simulink model "sim_2"  (R2020a)
settings: Solver=VariableStepAuto  StartTime=0.0  StopTime=10  MaxStep=0.2  RelTol=1e-3
values from neighbouring files (symbols this model uses):
  k1 = 50    [parameters.m]
  k2 = 20    [parameters.m]
  q0 = [0, 0]'    [parameters.m]
libraries: simulink x1
settings Model: Creator=sirius  LastModifiedBy=sirius

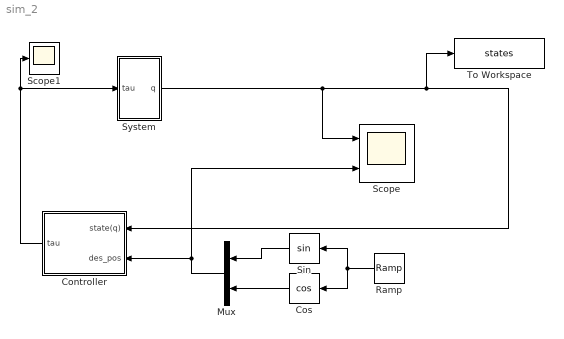
== system sim_2 ==
  Controller : Subsystem
  Cos : Trigonometry  Operator=cos
  Mux : Mux  Inputs=2
  Ramp : simulink/Sources/Ramp  slope=1  start=0  InitialOutput=0
  Scope : Scope  NumInputPorts=2
  Scope1 : Scope
  Sin : Trigonometry
  System : Subsystem
  To Workspace : ToWorkspace  VariableName=states  SampleTime=-1
  wires:
  Mux/1 -> Scope/2, Controller/2(des_pos)
  Controller/1(tau) -> Scope1/1, System/1(tau)
  System/1(q) -> Scope/1, To Workspace/1, Controller/1(state(q))
  Sin/1 -> Mux/1
  Cos/1 -> Mux/2
  Ramp/1 -> Sin/1, Cos/1

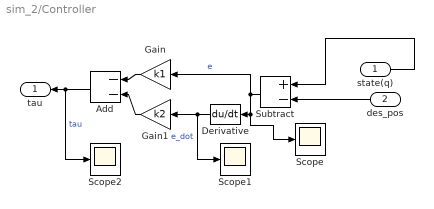
== system sim_2/Controller ==
  state(q) : Inport
  des_pos : Inport  Port=2
  Add : Sum  Inputs=--
  Derivative : Derivative
  Gain : Gain  Gain=k1
  Gain1 : Gain  Gain=k2
  Scope : Scope
  Scope1 : Scope
  Scope2 : Scope
  Subtract : Sum  Inputs=+-
  tau : Outport
  wires:
  Gain/1 -> Add/1
  state(q)/1 -> Subtract/1
  Gain1/1 -> Add/2
  Add/1 -> Scope2/1, tau/1  "tau"
  des_pos/1 -> Subtract/2
  Subtract/1 -> Gain/1, Scope/1, Derivative/1  "e"
  Derivative/1 -> Scope1/1, Gain1/1  "e_dot"

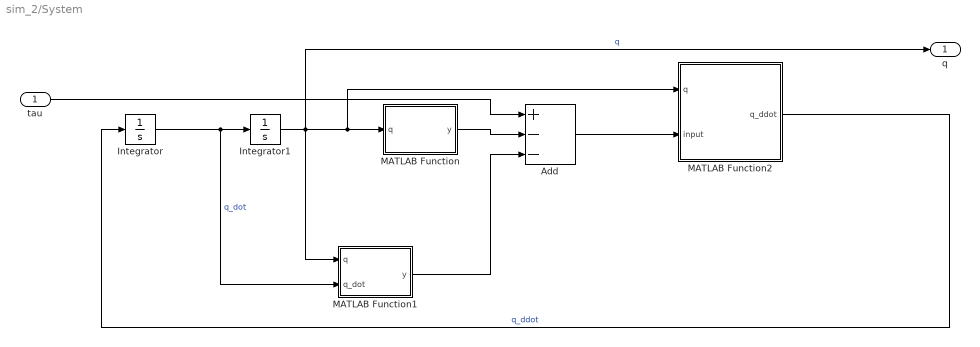
== system sim_2/System ==
  tau : Inport
  Add : Sum  Inputs=+--
  Integrator : Integrator  InitialCondition=q0
  Integrator1 : Integrator  InitialCondition=q0
  MATLAB Function : MATLAB Function  TreatAsAtomicUnit=on
  MATLAB Function1 : MATLAB Function  TreatAsAtomicUnit=on
  MATLAB Function2 : MATLAB Function  TreatAsAtomicUnit=on
  q : Outport
  wires:
  MATLAB Function1/1(y) -> Add/3
  Integrator1/1 -> MATLAB Function1/1(q), q/1, MATLAB Function2/1(q), MATLAB Function/1(q)  "q"
  tau/1 -> Add/1
  Integrator/1 -> MATLAB Function1/2(q_dot), Integrator1/1  "q_dot"
  MATLAB Function2/1(q_ddot) -> Integrator/1  "q_ddot"
  Add/1 -> MATLAB Function2/2(input)
  MATLAB Function/1(y) -> Add/2

== matlab function sim_2/System/MATLAB Function1 ==
  data: q input; y output; q_dot input
function y = V(q,q_dot)
y  = [-2*q_dot(1)*q_dot(2)*sin(q(2)) - (q_dot(2)^2)*sin(q(2));
      (q_dot(1)^2)*sin(q(2));
      ];

== matlab function sim_2/System/MATLAB Function2 ==
  data: q input; input input; q_ddot output
function q_ddot = M_inverse(q,input)
M = [3 + 2*cos(q(2)), 1 + cos(q(2));
    1 + cos(q(2)), 1;];
q_ddot = inv(M)*input;
% q_ddot = M/input;

== matlab function sim_2/System/MATLAB Function ==
  data: q input; y output
function y = G(q)
g = 9.81; %ms^-2
y = [2*g*cos(q(1)) + g*cos(q(1)+q(2));
     g*cos(q(1)+q(2));
     ];
